simulink model "MRAS_SMC_SFOC_1_5KW_15May21"  (R2017b)
settings: Solver=FixedStepDiscrete  StartTime=0.0  StopTime=3  FixedStep=Tsim  MaxStep=1e-6  RelTol=1e-3
values from neighbouring files (symbols this model uses):
  F = 1e-20    [ParametreMRAS_SMC_SFOC_1_5KW.m]
  Jm = 0.076    [ParametreMRAS_SMC_SFOC_1_5KW.m]
  Lm = 0.3032    [ParametreMRAS_SMC_SFOC_1_5KW.m]
  Lr = Lm+Lls    (= 0.32009)    [ParametreMRAS_SMC_SFOC_1_5KW.m]
  Ls = Lm+Llr    (= 0.32009)    [ParametreMRAS_SMC_SFOC_1_5KW.m]
  M = 0.3032    [ParametreMRAS_SMC_SFOC_1_5KW.m]
  Npole = 2    [ParametreMRAS_SMC_SFOC_1_5KW.m]
  Rr = 4.75    [ParametreMRAS_SMC_SFOC_1_5KW.m]
  Rs = 4.74    [ParametreMRAS_SMC_SFOC_1_5KW.m]
  sig = 1-((M^2)/(Ls*Lr))    (= 0.102748524929)    [ParametreMRAS_SMC_SFOC_1_5KW.m]
  T2_3 = T3_2'    [ParametreMRAS_SMC_SFOC_1_5KW.m]
  T3_2 = sqrt(2/3)*[cos(0) cos(2*pi/3) cos(4*pi/3);sin(0) sin(2*pi/3) sin(4*pi/3)]    [ParametreMRAS_SMC_SFOC_1_5KW.m]
  Tr = Lr/Rr    (= 0.0673873684211)    [ParametreMRAS_SMC_SFOC_1_5KW.m]
  Tsim = 0.5e-5    (= 5e-06)    [ParametreMRAS_SMC_SFOC_1_5KW.m]
  Tss = Ls/Rs    (= 0.067529535865)    [ParametreMRAS_SMC_SFOC_1_5KW.m]
undefined symbols (not defined in the file or in its folder): DiscIntNeverNeededParam
libraries: simulink x1
settings Model: Creator=momo  LastModifiedBy=LENOVO

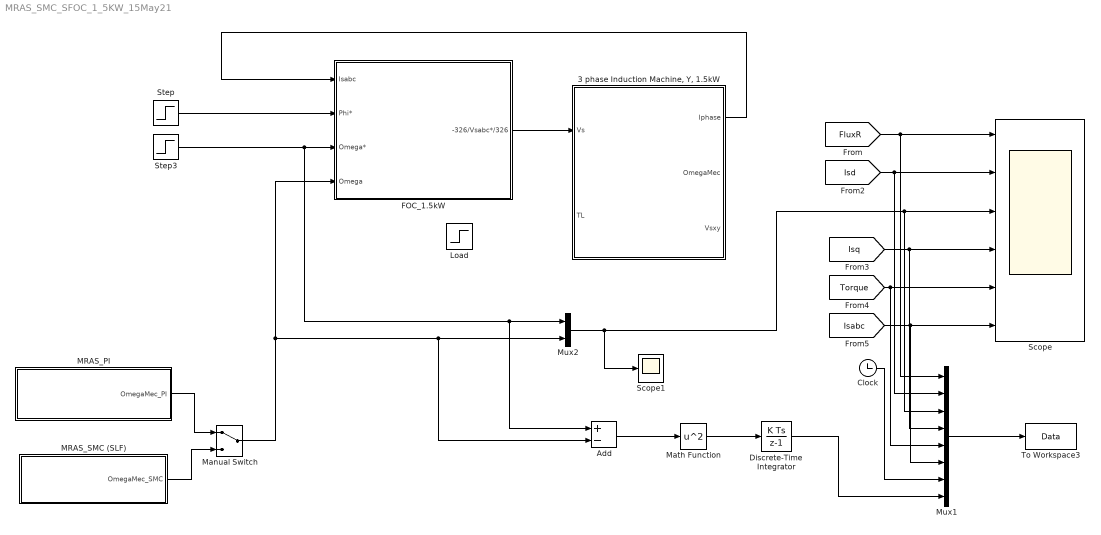
== system MRAS_SMC_SFOC_1_5KW_15May21 ==
  "3 phase Induction Machine, Y, 1.5kW" : Subsystem
  Add : Sum  Inputs=+-
  Clock : Clock
      settings: Decimation=100
  Discrete-Time Integrator : DiscreteIntegrator  InitialConditionSetting=State (most efficient)  SampleTime=-1  ICPrevOutput=DiscIntNeverNeededParam  ICPrevScaledInput=DiscIntNeverNeededParam
  FOC_1.5kW : Subsystem
  Load : Step  After=36.22  SampleTime=Tsim
  MRAS_PI : Subsystem
  MRAS_SMC (SLF) : Subsystem
  Manual Switch : ManualSwitch
  Math Function : Math  Operator=square  SaturateOnIntegerOverflow=on
  Mux1 : Mux  Inputs=8
  Mux2 : Mux  Inputs=2
  Scope : Scope  NumInputPorts=6
  Scope1 : Scope
  Step : Step  Time=0  After=1.2  SampleTime=Tsim
  Step3 : Step  Time=0.3  After=50  SampleTime=0
  To Workspace3 : ToWorkspace  VariableName=Data  SampleTime=-1
  wires:
  "3 phase Induction Machine, Y, 1.5kW"/1(Iphase) -> FOC_1.5kW/1(Isabc)
  Step/1 -> FOC_1.5kW/2(Phi*)
  [FluxR] -> Mux1/1, Scope/1
  [Isd] -> Mux1/2, Scope/2
  Mux2/1 -> Mux1/3, Scope/3, Scope1/1
  [Isq] -> Mux1/4, Scope/4
  [Torque] -> Mux1/5, Scope/5
  [Isabc] -> Mux1/6, Scope/6
  FOC_1.5kW/1(-326/Vsabc*/326) -> "3 phase Induction Machine, Y, 1.5kW"/1(Vs)
  Add/1 -> Math Function/1
  Math Function/1 -> Discrete-Time Integrator/1
  Step3/1 -> FOC_1.5kW/3(Omega*), Add/1, Mux2/1
  Manual Switch/1 -> Add/2, Mux2/2, FOC_1.5kW/4(Omega)
  Clock/1 -> Mux1/7
  Discrete-Time Integrator/1 -> Mux1/8
  Mux1/1 -> To Workspace3/1
  MRAS_SMC (SLF)/1(OmegaMec_SMC) -> Manual Switch/2
  MRAS_PI/1(OmegaMec_PI) -> Manual Switch/1

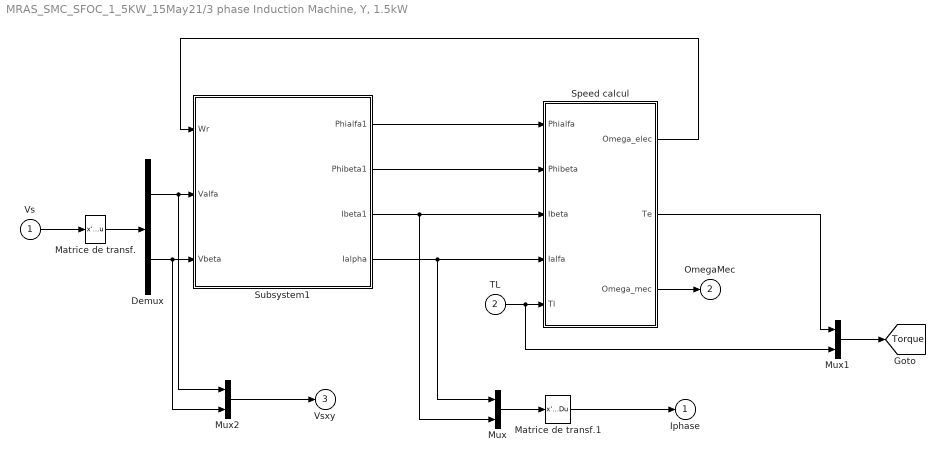
== system MRAS_SMC_SFOC_1_5KW_15May21/3 phase Induction Machine, Y, 1.5kW ==
  Vs : Inport
  TL : Inport  Port=2
  Demux : Demux  Outputs=2
  Matrice de transf. : StateSpace  A=[]  B=[]  C=[]  D=K  InitialCondition=0  mask(Matrix Gain){K=T3_2}
      mask prompts: K "Gain matrix:"
      mask help: Matrix Gain.
      mask Help: Multiplies input vector by entered matrix to produce output vector (y=Au).
      mask Display: disp('K')
  Matrice de transf.1 : StateSpace  A=[]  B=[]  C=[]  D=K  InitialCondition=0  mask(Matrix Gain){K=T2_3}
      mask prompts: K "Gain matrix:"
      mask help: Matrix Gain.
      mask Help: Multiplies input vector by entered matrix to produce output vector (y=Au).
      mask Display: disp('K')
  Mux : Mux  Inputs=2
  Mux1 : Mux  Inputs=2
  Mux2 : Mux  Inputs=2
  Speed calcul : Subsystem
  Subsystem1 : Subsystem
  Iphase : Outport  InitialOutput=0
  OmegaMec : Outport  Port=2  InitialOutput=0
  Vsxy : Outport  Port=3  InitialOutput=0
  tag scope: Torque=global
  wires:
  Subsystem1/3(Ibeta1) -> Speed calcul/3(Ibeta), Mux/2
  Subsystem1/4(Ialpha) -> Speed calcul/4(Ialfa), Mux/1
  Speed calcul/3(Omega_mec) -> OmegaMec/1
  Mux/1 -> Matrice de transf.1/1
  Matrice de transf./1 -> Demux/1
  Demux/2 -> Mux2/2, Subsystem1/3(Vbeta)
  Demux/1 -> Mux2/1, Subsystem1/2(Valfa)
  Subsystem1/2(Phibeta1) -> Speed calcul/2(Phibeta)
  Subsystem1/1(Phialfa1) -> Speed calcul/1(Phialfa)
  TL/1 -> Mux1/2, Speed calcul/5(Tl)
  Vs/1 -> Matrice de transf./1
  Matrice de transf.1/1 -> Iphase/1
  Speed calcul/1(Omega_elec) -> Subsystem1/1(Wr)
  Speed calcul/2(Te) -> Mux1/1
  Mux1/1 -> [Torque]
  Mux2/1 -> Vsxy/1

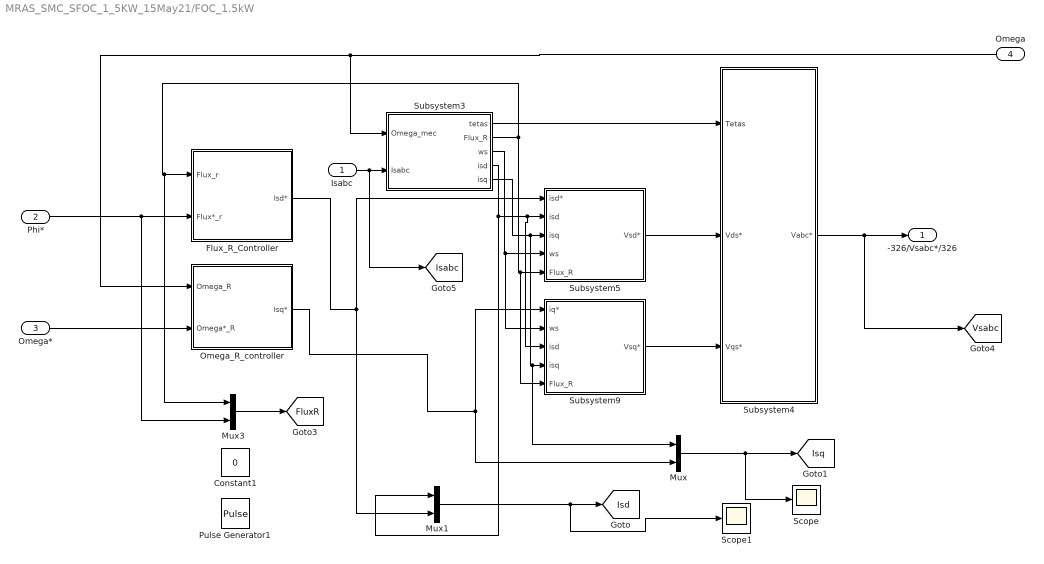
== system MRAS_SMC_SFOC_1_5KW_15May21/FOC_1.5kW ==
  Isabc : Inport
  Phi* : Inport  Port=2
  Omega* : Inport  Port=3
  Omega : Inport  Port=4
  Constant1 : Constant  Value=0
  Flux_R_Controller : Subsystem
  Mux : Mux  Inputs=2
  Mux1 : Mux  Inputs=2
  Mux3 : Mux  Inputs=2
  Omega_R_controller : Subsystem
  Pulse Generator1 : DiscretePulseGenerator  PulseType=Time based  Period=0.5  PulseWidth=50
  Scope : Scope
  Scope1 : Scope
  Subsystem3 : Subsystem
  Subsystem4 : Subsystem
  Subsystem5 : Subsystem
  Subsystem9 : Subsystem
  -326/Vsabc*/326 : Outport
  tag scope: FluxR=global, Isabc=global, Isd=global, Isq=global, Vsabc=global
  wires:
  Subsystem4/1(Vabc*) -> [Vsabc], -326/Vsabc*/326/1
  Omega/1 -> Omega_R_controller/1(Omega_R), Subsystem3/1(Omega_mec)
  Omega*/1 -> Omega_R_controller/2(Omega*_R)
  Isabc/1 -> [Isabc], Subsystem3/2(Isabc)
  Mux/1 -> Scope/1, [Isq]
  Mux1/1 -> Scope1/1, [Isd]
  Subsystem5/1(Vsd*) -> Subsystem4/2(Vds*)
  Subsystem9/1(Vsq*) -> Subsystem4/3(Vqs*)
  Phi*/1 -> Mux3/2, Flux_R_Controller/2(Flux*_r)
  Subsystem3/1(tetas) -> Subsystem4/1(Tetas)
  Subsystem3/3(ws) -> Subsystem9/2(ws), Subsystem5/4(ws)
  Subsystem3/4(isd) -> Mux1/1, Subsystem9/3(isd), Subsystem5/2(isd)
  Subsystem3/5(isq) -> Mux/1, Subsystem9/4(isq), Subsystem5/3(isq)
  Subsystem3/2(Flux_R) -> Subsystem9/5(Flux_R), Subsystem5/5(Flux_R), Mux3/1, Flux_R_Controller/1(Flux_r)
  Mux3/1 -> [FluxR]
  Omega_R_controller/1(Isq*) -> Mux/2, Subsystem9/1(iq*)
  Flux_R_Controller/1(Isd*) -> Mux1/2, Subsystem5/1(isd*)

== system MRAS_SMC_SFOC_1_5KW_15May21/MRAS_PI ==
  Gain1 : Gain  Gain=60/2/pi/2
  PI : simulink/Continuous/PID Controller  Controller=PID  TimeDomain=Discrete-time  SampleTime=Tsim  IntegratorMethod=Forward Euler  FilterMethod=Forward Euler  Form=Parallel  UseFilter=on  ControllerParametersSource=internal  P=200  I=4000  D=0  N=100  InitialConditionSource=internal  InitialConditionForIntegrator=0  InitialConditionForFilter=0  ExternalReset=none  LimitOutput=on  UpperSaturationLimit=400  LowerSaturationLimit=-400  LinearizeAsGain=off  AntiWindupMode=none  Kb=1  TrackingMode=off  Kt=1  PParamMin=[]  PParamMax=[]  IParamMin=[]  IParamMax=[]  DParamMin=[]  DParamMax=[]  NParamMin=[]  NParamMax=[]  KbParamMin=[]  KbParamMax=[]  KtParamMin=[]  KtParamMax=[]  POutMin=[]  POutMax=[]  IOutMin=[]  IOutMax=[]  DOutMin=[]  DOutMax=[]  NOutMin=[]  NOutMax=[]  KbOutMin=[]  KbOutMax=[]  KtOutMin=[]  KtOutMax=[]  IntegratorOutMin=[]  IntegratorOutMax=[]  FilterOutMin=[]  FilterOutMax=[]  SumOutMin=[]  SumOutMax=[]  SumI1OutMin=[]  SumI1OutMax=[]  SumI2OutMin=[]  SumI2OutMax=[]  SumI3OutMin=[]  SumI3OutMax=[]  SumDOutMin=[]  SumDOutMax=[]  SaturationOutMin=[]  SaturationOutMax=[]  IntegratorContinuousStateAttributes=''  IntegratorStateMustResolveToSignalObject=off  IntegratorRTWStateStorageClass=Auto  FilterContinuousStateAttributes=''  FilterStateMustResolveToSignalObject=off  FilterRTWStateStorageClass=Auto  DifferentiatorICPrevScaledInput=0  DifferentiatorOutMin=[]  DifferentiatorOutMax=[]  InitialConditionSetting=State (most efficient)  FilterDiffOutCoefMin=[]  FilterDiffOutCoefMax=[]  SumDenOutMin=[]  SumDenOutMax=[]  SumNumOutMin=[]  SumNumOutMax=[]  ReciprocalOutMin=[]  ReciprocalOutMax=[]  DivideOutMin=[]  DivideOutMax=[]  TunerSelectOption=Transfer Function Based (PID Tuner App)
  Product1 : Product  RndMeth=Zero
  Product2 : Product  RndMeth=Zero
  Subsystem1 : Subsystem
  Subtract1 : Sum  Inputs=-+
  OmegaMec_PI : Outport
  wires:
  Subtract1/1 -> PI/1
  PI/1 -> Gain1/1, Subsystem1/3(wr)
  Product2/1 -> Subtract1/2
  Product1/1 -> Subtract1/1
  [Vsabc] -> Subsystem1/2(Vphase)
  [Isabc] -> Subsystem1/1(iphase)
  Subsystem1/3(phi_r_al_esti) -> Product2/2
  Subsystem1/2(phi_r_beta_ref) -> Product2/1
  Subsystem1/4(phi_r_beta_estim) -> Product1/2
  Subsystem1/1(phi_r_al_ref) -> Product1/1
  Gain1/1 -> OmegaMec_PI/1

== system MRAS_SMC_SFOC_1_5KW_15May21/MRAS_SMC (SLF) ==
  Gain1 : Gain  Gain=60/2/pi/2
  Product1 : Product  RndMeth=Zero
  Product2 : Product  RndMeth=Zero
  Subsystem1 : Subsystem
  Subsystem6 : Subsystem
  Subtract1 : Sum  Inputs=-+
  OmegaMec_SMC : Outport
  wires:
  [Vsabc] -> Subsystem1/2(Vphase)
  [Isabc] -> Subsystem1/1(iphase)
  Gain1/1 -> OmegaMec_SMC/1
  Subtract1/1 -> Subsystem6/1(Error)
  Subsystem6/1(Wm) -> Gain1/1, Subsystem1/3(wr)
  Product2/1 -> Subtract1/2
  Product1/1 -> Subtract1/1
  Subsystem1/3(phi_r_al_esti) -> Product2/2
  Subsystem1/2(phi_r_beta_ref) -> Product2/1
  Subsystem1/4(phi_r_beta_estim) -> Product1/2
  Subsystem1/1(phi_r_al_ref) -> Product1/1

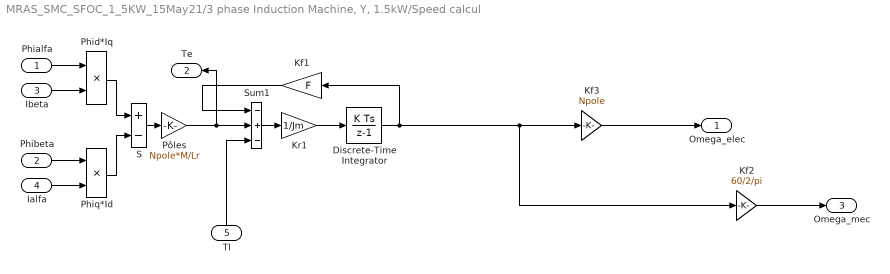
== system MRAS_SMC_SFOC_1_5KW_15May21/3 phase Induction Machine, Y, 1.5kW/Speed calcul ==
  Phialfa : Inport
  Phibeta : Inport  Port=2
  Ibeta : Inport  Port=3
  Ialfa : Inport  Port=4
  Tl : Inport  Port=5
  Discrete-Time Integrator : DiscreteIntegrator  InitialConditionSetting=State (most efficient)  SampleTime=Tsim  ICPrevOutput=DiscIntNeverNeededParam  ICPrevScaledInput=DiscIntNeverNeededParam
  Kf1 : Gain  Gain=F  OutDataTypeStr=Inherit: Same as input  ParamDataTypeStr=Inherit: Same as input
  Kf2 : Gain  Gain=60/2/pi  SaturateOnIntegerOverflow=on  OutDataTypeStr=Inherit: Same as input  ParamDataTypeStr=Inherit: Same as input
  Kf3 : Gain  Gain=Npole  SaturateOnIntegerOverflow=on  OutDataTypeStr=Inherit: Same as input  ParamDataTypeStr=Inherit: Same as input
  Kr1 : Gain  Gain=1/Jm  OutDataTypeStr=Inherit: Same as input  ParamDataTypeStr=Inherit: Same as input
  Phid*Iq : Product  SaturateOnIntegerOverflow=on  RndMeth=Zero  InputSameDT=on  OutDataTypeStr=Inherit: Same as first input
  Phiq*Id : Product  SaturateOnIntegerOverflow=on  RndMeth=Zero  InputSameDT=on  OutDataTypeStr=Inherit: Same as first input
  Pôles : Gain  Gain=Npole*M/Lr  SaturateOnIntegerOverflow=on  OutDataTypeStr=Inherit: Same as input  ParamDataTypeStr=Inherit: Same as input
  S : Sum  Inputs=+-  SaturateOnIntegerOverflow=on  InputSameDT=on  OutDataTypeStr=Inherit: Same as first input
  Sum1 : Sum  Inputs=-+-  InputSameDT=on  OutDataTypeStr=Inherit: Same as first input
  Omega_elec : Outport
  Te : Outport  Port=2
  Omega_mec : Outport  Port=3
  wires:
  Kf2/1 -> Omega_mec/1
  Tl/1 -> Sum1/3
  Phibeta/1 -> Phiq*Id/1
  Kf3/1 -> Omega_elec/1
  Ialfa/1 -> Phiq*Id/2
  Ibeta/1 -> Phid*Iq/2
  Phialfa/1 -> Phid*Iq/1
  Phiq*Id/1 -> S/2
  Phid*Iq/1 -> S/1
  Discrete-Time Integrator/1 -> Kf3/1, Kf2/1, Kf1/1
  Kr1/1 -> Discrete-Time Integrator/1
  Sum1/1 -> Kr1/1
  Pôles/1 -> Te/1, Sum1/2
  S/1 -> Pôles/1
  Kf1/1 -> Sum1/1

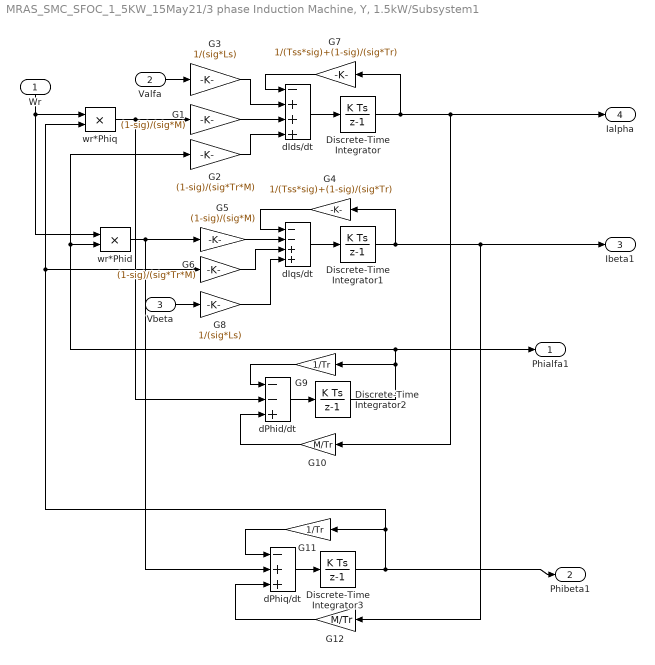
== system MRAS_SMC_SFOC_1_5KW_15May21/3 phase Induction Machine, Y, 1.5kW/Subsystem1 ==
  Wr : Inport
  Valfa : Inport  Port=2
  Vbeta : Inport  Port=3
  Discrete-Time Integrator{,1..3} (4 alike) : DiscreteIntegrator  InitialConditionSetting=State (most efficient)  SampleTime=Tsim  ICPrevOutput=DiscIntNeverNeededParam  ICPrevScaledInput=DiscIntNeverNeededParam
  G1 : Gain  Gain=(1-sig)/(sig*M)  SaturateOnIntegerOverflow=on  OutDataTypeStr=Inherit: Same as input  ParamDataTypeStr=Inherit: Same as input
  G10 : Gain  Gain=M/Tr  SaturateOnIntegerOverflow=on  OutDataTypeStr=Inherit: Same as input  ParamDataTypeStr=Inherit: Same as input
  G11 : Gain  Gain=1/Tr  SaturateOnIntegerOverflow=on  OutDataTypeStr=Inherit: Same as input  ParamDataTypeStr=Inherit: Same as input
  G12 : Gain  Gain=M/Tr  SaturateOnIntegerOverflow=on  OutDataTypeStr=Inherit: Same as input  ParamDataTypeStr=Inherit: Same as input
  G2 : Gain  Gain=(1-sig)/(sig*Tr*M)  SaturateOnIntegerOverflow=on  OutDataTypeStr=Inherit: Same as input  ParamDataTypeStr=Inherit: Same as input
  G3 : Gain  Gain=1/(sig*Ls)  SaturateOnIntegerOverflow=on  OutDataTypeStr=Inherit: Same as input  ParamDataTypeStr=Inherit: Same as input
  G4 : Gain  Gain=1/(Tss*sig)+(1-sig)/(sig*Tr)  SaturateOnIntegerOverflow=on  OutDataTypeStr=Inherit: Same as input  ParamDataTypeStr=Inherit: Same as input
  G5 : Gain  Gain=(1-sig)/(sig*M)  SaturateOnIntegerOverflow=on  OutDataTypeStr=Inherit: Same as input  ParamDataTypeStr=Inherit: Same as input
  G6 : Gain  Gain=(1-sig)/(sig*Tr*M)  SaturateOnIntegerOverflow=on  OutDataTypeStr=Inherit: Same as input  ParamDataTypeStr=Inherit: Same as input
  G7 : Gain  Gain=1/(Tss*sig)+(1-sig)/(sig*Tr)  SaturateOnIntegerOverflow=on  OutDataTypeStr=Inherit: Same as input  ParamDataTypeStr=Inherit: Same as input
  G8 : Gain  Gain=1/(sig*Ls)  SaturateOnIntegerOverflow=on  OutDataTypeStr=Inherit: Same as input  ParamDataTypeStr=Inherit: Same as input
  G9 : Gain  Gain=1/Tr  SaturateOnIntegerOverflow=on  OutDataTypeStr=Inherit: Same as input  ParamDataTypeStr=Inherit: Same as input
  dIds/dt : Sum  Inputs=-+++  SaturateOnIntegerOverflow=on  InputSameDT=on  OutDataTypeStr=Inherit: Same as first input
  dIqs/dt : Sum  Inputs=--++  SaturateOnIntegerOverflow=on  InputSameDT=on  OutDataTypeStr=Inherit: Same as first input
  dPhid/dt : Sum  Inputs=--+  SaturateOnIntegerOverflow=on  InputSameDT=on  OutDataTypeStr=Inherit: Same as first input
  dPhiq/dt : Sum  Inputs=-++  SaturateOnIntegerOverflow=on  InputSameDT=on  OutDataTypeStr=Inherit: Same as first input
  wr*Phid : Product  SaturateOnIntegerOverflow=on  RndMeth=Zero  InputSameDT=on  OutDataTypeStr=Inherit: Same as first input
  wr*Phiq : Product  SaturateOnIntegerOverflow=on  RndMeth=Zero  InputSameDT=on  OutDataTypeStr=Inherit: Same as first input
  Phialfa1 : Outport
  Phibeta1 : Outport  Port=2
  Ibeta1 : Outport  Port=3
  Ialpha : Outport  Port=4
  wires:
  Vbeta/1 -> G8/1
  Valfa/1 -> G3/1
  Wr/1 -> wr*Phiq/1, wr*Phid/1
  dIds/dt/1 -> Discrete-Time Integrator/1
  Discrete-Time Integrator/1 -> G10/1, Ialpha/1, G7/1
  G7/1 -> dIds/dt/1
  G1/1 -> dIds/dt/3
  G3/1 -> dIds/dt/2
  G2/1 -> dIds/dt/4
  dPhid/dt/1 -> Discrete-Time Integrator2/1
  Discrete-Time Integrator2/1 -> G9/1, Phialfa1/1, G2/1, wr*Phid/2
  G9/1 -> dPhid/dt/1
  G10/1 -> dPhid/dt/3
  G11/1 -> dPhiq/dt/1
  G12/1 -> dPhiq/dt/3
  G8/1 -> dIqs/dt/4
  G6/1 -> dIqs/dt/3
  G5/1 -> dIqs/dt/2
  wr*Phid/1 -> G5/1, dPhiq/dt/2
  G4/1 -> dIqs/dt/1
  Discrete-Time Integrator1/1 -> G12/1, Ibeta1/1, G4/1
  wr*Phiq/1 -> G1/1, dPhid/dt/2
  Discrete-Time Integrator3/1 -> G6/1, wr*Phiq/2, G11/1, Phibeta1/1
  dPhiq/dt/1 -> Discrete-Time Integrator3/1
  dIqs/dt/1 -> Discrete-Time Integrator1/1

== system MRAS_SMC_SFOC_1_5KW_15May21/FOC_1.5kW/Flux_R_Controller ==
  Flux_r : Inport
  Flux*_r : Inport  Port=2
  -5<isd*<5 : Saturate  UpperLimit=5  LowerLimit=-5
  Add1 : Sum  Inputs=-+
  Add2 : Sum
  Gain : Gain  Gain=1000
  Gain1 : Gain  Gain=100
  Saturated_Integrator : DiscreteIntegrator  InitialConditionSetting=State (most efficient)  SampleTime=Tsim  LimitOutput=on  UpperSaturationLimit=5  LowerSaturationLimit=-5  ICPrevOutput=DiscIntNeverNeededParam  ICPrevScaledInput=DiscIntNeverNeededParam
  Scope : Scope
  Isd* : Outport
  wires:
  Gain/1 -> Saturated_Integrator/1
  Gain1/1 -> Add2/2
  Add2/1 -> -5<isd*<5/1
  Saturated_Integrator/1 -> Scope/1, Add2/1
  -5<isd*<5/1 -> Isd*/1
  Flux_r/1 -> Add1/1
  Flux*_r/1 -> Add1/2
  Add1/1 -> Gain1/1, Gain/1

== system MRAS_SMC_SFOC_1_5KW_15May21/FOC_1.5kW/Omega_R_controller ==
  Omega_R : Inport
  Omega*_R : Inport  Port=2
  -5<isq*<5 : Saturate  UpperLimit=5  LowerLimit=-5
  Add : Sum  Inputs=-+
  Add2 : Sum
  Discrete-Time Integrator : DiscreteIntegrator  InitialConditionSetting=State (most efficient)  SampleTime=Tsim  LimitOutput=on  UpperSaturationLimit=5  LowerSaturationLimit=-5  ICPrevOutput=DiscIntNeverNeededParam  ICPrevScaledInput=DiscIntNeverNeededParam
  Gain1 : Gain  Gain=10
  Gain3 : Gain  Gain=0
  Gain4 : Gain  Gain=100
  Kf1 : Gain  Gain=2*pi/60  SaturateOnIntegerOverflow=on  OutDataTypeStr=Inherit: Same as input  ParamDataTypeStr=Inherit: Same as input
  Scope : Scope
  Isq* : Outport
  wires:
  -5<isq*<5/1 -> Scope/1, Isq*/1
  Discrete-Time Integrator/1 -> Add2/1
  Add2/1 -> -5<isq*<5/1
  Gain1/1 -> Add2/2
  Gain3/1 -> Discrete-Time Integrator/1
  Omega*_R/1 -> Add/2
  Omega_R/1 -> Add/1
  Add/1 -> Kf1/1
  Kf1/1 -> Gain3/1, Gain1/1

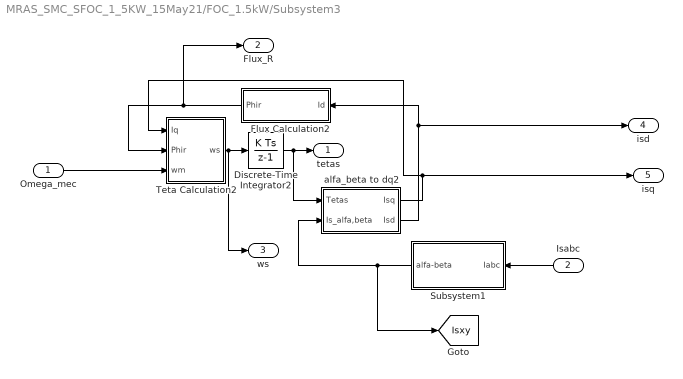
== system MRAS_SMC_SFOC_1_5KW_15May21/FOC_1.5kW/Subsystem3 ==
  Omega_mec : Inport
  Isabc : Inport  Port=2
  Discrete-Time Integrator2 : DiscreteIntegrator  InitialConditionSetting=State (most efficient)  SampleTime=Tsim  ICPrevOutput=DiscIntNeverNeededParam  ICPrevScaledInput=DiscIntNeverNeededParam
  Flux Calculation2 : Subsystem  mask(Flux Calcultation){}
      mask init:
      | NF=0.44572610323020e-6;
      | DF=[1 -0.99998715486734];
      mask Display: disp('Flux\nCalc.')
  Subsystem1 : Subsystem
  Teta Calculation2 : Subsystem
  alfa_beta to dq2 : Subsystem
  tetas : Outport
  Flux_R : Outport  Port=2
  ws : Outport  Port=3
  isd : Outport  Port=4
  isq : Outport  Port=5
  tag scope: Isxy=global
  wires:
  Teta Calculation2/1(ws) -> Discrete-Time Integrator2/1, ws/1
  alfa_beta to dq2/1(Isq) -> Teta Calculation2/1(Iq), isq/1
  alfa_beta to dq2/2(Isd) -> Flux Calculation2/1(Id), isd/1
  Discrete-Time Integrator2/1 -> tetas/1, alfa_beta to dq2/1(Tetas)
  Flux Calculation2/1(Phir) -> Teta Calculation2/2(Phir), Flux_R/1
  Subsystem1/1(alfa-beta) -> [Isxy], alfa_beta to dq2/2(Is_alfa,beta)
  Isabc/1 -> Subsystem1/1(Iabc)
  Omega_mec/1 -> Teta Calculation2/3(wm)

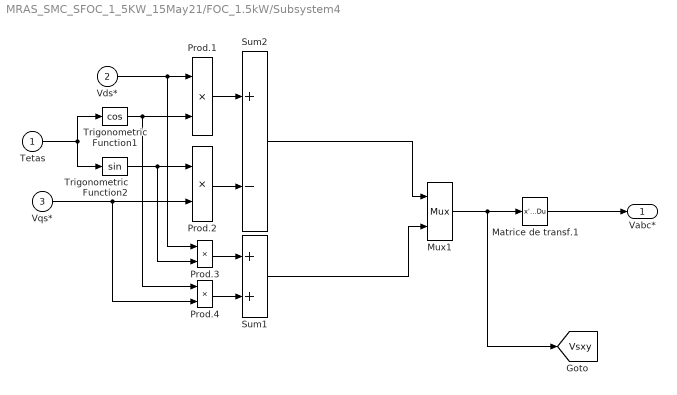
== system MRAS_SMC_SFOC_1_5KW_15May21/FOC_1.5kW/Subsystem4 ==
  Tetas : Inport
  Vds* : Inport  Port=2
  Vqs* : Inport  Port=3
  Matrice de transf.1 : StateSpace  A=[]  B=[]  C=[]  D=K  InitialCondition=0  mask(Matrix Gain){K=T2_3}
      mask prompts: K "Gain matrix:"
      mask help: Matrix Gain.
      mask Help: Multiplies input vector by entered matrix to produce output vector (y=Au).
      mask Display: disp('K')
  Mux1 : Mux  Inputs=2
  Prod.{1..4} (4 alike) : Product  SaturateOnIntegerOverflow=on  InputSameDT=on  OutDataTypeStr=Inherit: Same as first input
  Sum1 : Sum  SaturateOnIntegerOverflow=on  InputSameDT=on  OutDataTypeStr=Inherit: Same as first input
  Sum2 : Sum  Inputs=+-  SaturateOnIntegerOverflow=on  InputSameDT=on  OutDataTypeStr=Inherit: Same as first input
  Trigonometric Function1 : Trigonometry  Operator=cos
  Trigonometric Function2 : Trigonometry
  Vabc* : Outport
  tag scope: Vsxy=global
  wires:
  Tetas/1 -> Trigonometric Function1/1, Trigonometric Function2/1
  Prod.4/1 -> Sum1/2
  Prod.3/1 -> Sum1/1
  Vqs*/1 -> Prod.2/2, Prod.4/2
  Vds*/1 -> Prod.1/1, Prod.3/1
  Prod.2/1 -> Sum2/2
  Prod.1/1 -> Sum2/1
  Trigonometric Function2/1 -> Prod.3/2, Prod.2/1
  Trigonometric Function1/1 -> Prod.4/1, Prod.1/2
  Mux1/1 -> [Vsxy], Matrice de transf.1/1
  Sum1/1 -> Mux1/2
  Matrice de transf.1/1 -> Vabc*/1
  Sum2/1 -> Mux1/1

== system MRAS_SMC_SFOC_1_5KW_15May21/FOC_1.5kW/Subsystem5 ==
  isd* : Inport
  isd : Inport  Port=2
  isq : Inport  Port=3
  ws : Inport  Port=4
  Flux_R : Inport  Port=5
  -400<Vsd*<400 : Saturate  UpperLimit=400  LowerLimit=-400
  Add : Sum  Inputs=-+
  Add4 : Sum  Inputs=+-
  Mux2 : Mux  Inputs=3
  d-Current controller : Subsystem
  femd : Fcn  Expr=u(3)*sig*Ls*u(1)+(M/Lr^2)*Rr*u(2)
  Vsd* : Outport  InitialOutput=0
  wires:
  isd/1 -> Add/1
  isd*/1 -> Add/2
  Mux2/1 -> femd/1
  isq/1 -> Mux2/1
  ws/1 -> Mux2/3
  Flux_R/1 -> Mux2/2
  Add4/1 -> -400<Vsd*<400/1
  -400<Vsd*<400/1 -> Vsd*/1
  femd/1 -> Add4/2
  Add/1 -> d-Current controller/1(Error Isd)
  d-Current controller/1(Vsd*) -> Add4/1

== system MRAS_SMC_SFOC_1_5KW_15May21/FOC_1.5kW/Subsystem9 ==
  iq* : Inport
  ws : Inport  Port=2
  isd : Inport  Port=3
  isq : Inport  Port=4
  Flux_R : Inport  Port=5
  -400<V*sq<400 : Saturate  UpperLimit=400  LowerLimit=-400
  Add : Sum  Inputs=-+
  Add3 : Sum  Inputs=+-
  Fcn1 : Fcn  Expr=-u(4)*sig*Ls*u(1)-u(4)*(M/Lr)*u(3)+(M^2/Lr/Tr)*u(2)
  Mux1 : Mux
  q-Current controller : Subsystem
  Vsq* : Outport  InitialOutput=0
  wires:
  Mux1/1 -> Fcn1/1
  ws/1 -> Mux1/4
  isd/1 -> Mux1/1
  Flux_R/1 -> Mux1/3
  isq/1 -> Mux1/2, Add/1
  iq*/1 -> Add/2
  Add3/1 -> -400<V*sq<400/1
  -400<V*sq<400/1 -> Vsq*/1
  Fcn1/1 -> Add3/2
  Add/1 -> q-Current controller/1(Error Isq)
  q-Current controller/1(Vsq*) -> Add3/1

== system MRAS_SMC_SFOC_1_5KW_15May21/MRAS_PI/Subsystem1 ==
  iphase : Inport
  Vphase : Inport  Port=2
  wr : Inport  Port=3
  Subsystem : Subsystem
  model reference : Subsystem
  phi_r_al_ref : Outport
  phi_r_beta_ref : Outport  Port=2
  phi_r_al_esti : Outport  Port=3
  phi_r_beta_estim : Outport  Port=4
  wires:
  model reference/2(phi_r_bet_ref) -> phi_r_beta_ref/1
  model reference/1(phi_r_al_ref) -> phi_r_al_ref/1
  iphase/1 -> model reference/1(Iaa'bb'cc')
  Vphase/1 -> model reference/2(Vaa'bb'cc')
  Subsystem/2(PhirBeta) -> phi_r_beta_estim/1
  Subsystem/1(Phiralpha) -> phi_r_al_esti/1
  model reference/3(Isal) -> Subsystem/1(Isalpha)
  model reference/4(Isbeta) -> Subsystem/2(Isbeta)
  wr/1 -> Subsystem/3(In3)

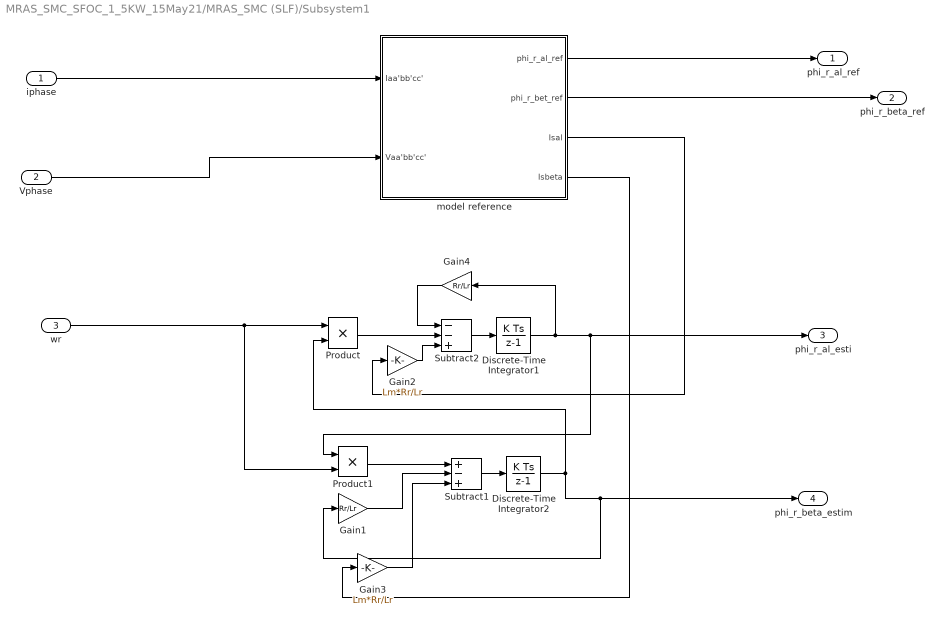
== system MRAS_SMC_SFOC_1_5KW_15May21/MRAS_SMC (SLF)/Subsystem1 ==
  iphase : Inport
  Vphase : Inport  Port=2
  wr : Inport  Port=3
  Discrete-Time Integrator1 : DiscreteIntegrator  InitialConditionSetting=State (most efficient)  SampleTime=Tsim  ICPrevOutput=DiscIntNeverNeededParam  ICPrevScaledInput=DiscIntNeverNeededParam
  Discrete-Time Integrator2 : DiscreteIntegrator  InitialConditionSetting=State (most efficient)  SampleTime=Tsim  ICPrevOutput=DiscIntNeverNeededParam  ICPrevScaledInput=DiscIntNeverNeededParam
  Gain1 : Gain  Gain=Rr/Lr
  Gain2 : Gain  Gain=Lm*Rr/Lr
  Gain3 : Gain  Gain=Lm*Rr/Lr
  Gain4 : Gain  Gain=Rr/Lr
  Product : Product  RndMeth=Zero
  Product1 : Product  RndMeth=Zero
  Subtract1 : Sum  Inputs=+-+
  Subtract2 : Sum  Inputs=--+
  model reference : Subsystem
  phi_r_al_ref : Outport
  phi_r_beta_ref : Outport  Port=2
  phi_r_al_esti : Outport  Port=3
  phi_r_beta_estim : Outport  Port=4
  wires:
  Subtract2/1 -> Discrete-Time Integrator1/1
  Discrete-Time Integrator1/1 -> phi_r_al_esti/1, Product1/1, Gain4/1
  Vphase/1 -> model reference/2(Vaa'bb'cc')
  iphase/1 -> model reference/1(Iaa'bb'cc')
  model reference/1(phi_r_al_ref) -> phi_r_al_ref/1
  model reference/2(phi_r_bet_ref) -> phi_r_beta_ref/1
  Subtract1/1 -> Discrete-Time Integrator2/1
  Discrete-Time Integrator2/1 -> Product/2, phi_r_beta_estim/1, Gain1/1
  Product/1 -> Subtract2/2
  wr/1 -> Product/1, Product1/2
  Product1/1 -> Subtract1/1
  Gain2/1 -> Subtract2/3
  Gain3/1 -> Subtract1/3
  Gain4/1 -> Subtract2/1
  Gain1/1 -> Subtract1/2
  model reference/4(Isbeta) -> Gain3/1
  model reference/3(Isal) -> Gain2/1

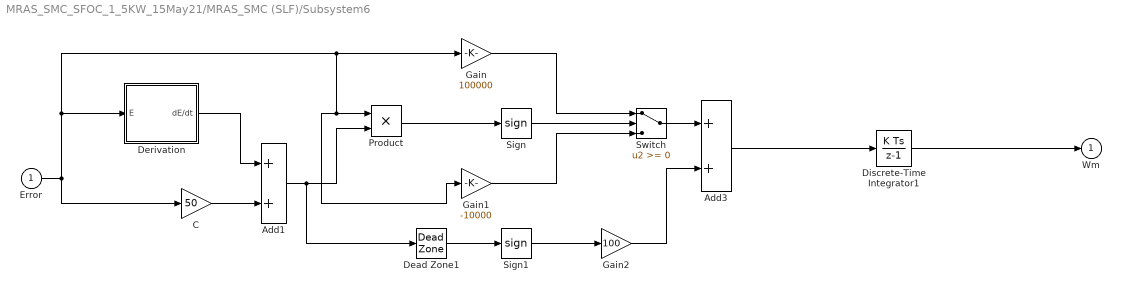
== system MRAS_SMC_SFOC_1_5KW_15May21/MRAS_SMC (SLF)/Subsystem6 ==
  Error : Inport
  Add1 : Sum
  Add3 : Sum
  C : Gain  Gain=50
  Dead Zone1 : DeadZone  LowerValue=-.3  UpperValue=.3  SaturateOnIntegerOverflow=on
  Derivation : Subsystem
  Discrete-Time Integrator1 : DiscreteIntegrator  InitialConditionSetting=State (most efficient)  SampleTime=Tsim  ICPrevOutput=DiscIntNeverNeededParam  ICPrevScaledInput=DiscIntNeverNeededParam
  Gain : Gain  Gain=100000
  Gain1 : Gain  Gain=-10000
  Gain2 : Gain  Gain=100
  Product : Product  RndMeth=Zero
  Sign : Signum
  Sign1 : Signum  ZeroCross=off
  Switch : Switch
  Wm : Outport  InitialOutput=0
  wires:
  Gain2/1 -> Add3/2
  Dead Zone1/1 -> Sign1/1
  Derivation/1(dE/dt) -> Add1/1
  Discrete-Time Integrator1/1 -> Wm/1
  Add1/1 -> Product/2, Dead Zone1/1
  Sign1/1 -> Gain2/1
  Gain1/1 -> Switch/3
  Gain/1 -> Switch/1
  Add3/1 -> Discrete-Time Integrator1/1
  Switch/1 -> Add3/1
  Sign/1 -> Switch/2
  Product/1 -> Sign/1
  Error/1 -> C/1, Gain1/1, Product/1, Gain/1, Derivation/1(E)
  C/1 -> Add1/2

== system MRAS_SMC_SFOC_1_5KW_15May21/FOC_1.5kW/Subsystem3/Flux Calculation2 ==
  Id : Inport
  Discrete Tranfer Function1 : Subsystem  mask(First Order Low Pass Filter (Discrete)){T=Tr, Ts=Tsim}
      mask prompts: T "Time constant T (s) :"; Ts "Time step (s)"
      mask help: H(s)=1/(1+T.s)
      mask init:
      | X=[0 1 2 3 4];
      |  Y=[-2 -2 -3 -4 -4];
      |  str=sprintf('\nH=1/(1+T.s)\n T= %g s\n\n\n',T);
      | num=1;
      | den=[T 1];
      | 
      | % discrete transfer function
      | % descending powers of z
      | numd= Ts/T;
      | dend=[ 1  (Ts-T)/T];
      mask Display:
      | plot(X,Y);
      | disp(str);
  M1 : Gain  Gain=M  SaturateOnIntegerOverflow=on  OutDataTypeStr=Inherit: Same as input  ParamDataTypeStr=Inherit: Same as input
  Phir : Outport
  wires:
  Id/1 -> Discrete Tranfer Function1/1(In)
  M1/1 -> Phir/1
  Discrete Tranfer Function1/1(Out) -> M1/1

== system MRAS_SMC_SFOC_1_5KW_15May21/FOC_1.5kW/Subsystem3/Subsystem1 ==
  Iabc : Inport
  Matrice2 : StateSpace  A=[]  B=[]  C=[]  D=K  InitialCondition=0  mask(Matrix Gain){K=T3_2}
      mask prompts: K "Gain matrix:"
      mask help: Matrix Gain.
      mask Help: Multiplies input vector by entered matrix to produce output vector (y=Au).
      mask Display: disp('K')
  alfa-beta : Outport
  wires:
  Iabc/1 -> Matrice2/1
  Matrice2/1 -> alfa-beta/1

== system MRAS_SMC_SFOC_1_5KW_15May21/FOC_1.5kW/Subsystem3/Teta Calculation2 ==
  Iq : Inport
  Phir : Inport  Port=2
  wm : Inport  Port=3
  Fcn : Fcn  Expr=M*u(1)/(u(2)*Tr+1e-12)
  Gain2 : Gain  SaturateOnIntegerOverflow=on  OutDataTypeStr=Inherit: Same as input  ParamDataTypeStr=Inherit: Same as input
  Kf1 : Gain  Gain=Npole  SaturateOnIntegerOverflow=on  OutDataTypeStr=Inherit: Same as input  ParamDataTypeStr=Inherit: Same as input
  Kf2 : Gain  Gain=2*pi/60  SaturateOnIntegerOverflow=on  OutDataTypeStr=Inherit: Same as input  ParamDataTypeStr=Inherit: Same as input
  Mux : Mux  Inputs=2
  Scope : Scope
  Sum : Sum  SaturateOnIntegerOverflow=on  InputSameDT=on  OutDataTypeStr=Inherit: Same as first input
  ws : Outport  InitialOutput=0
  tag scope: wsl=global
  wires:
  Kf1/1 -> Kf2/1
  Mux/1 -> Fcn/1
  Iq/1 -> Mux/1
  Phir/1 -> Scope/1, Mux/2
  Fcn/1 -> Gain2/1
  wm/1 -> Kf1/1
  Sum/1 -> ws/1
  Kf2/1 -> Sum/2
  Gain2/1 -> [wsl], Sum/1

== system MRAS_SMC_SFOC_1_5KW_15May21/FOC_1.5kW/Subsystem3/alfa_beta to dq2 ==
  Tetas : Inport
  Is_alfa,beta : Inport  Port=2
  Fcn : Fcn  Expr=sin(u)
  Fcn1 : Fcn  Expr=cos(u)
  Gain : Gain  OutDataTypeStr=Inherit: Same as input  ParamDataTypeStr=Inherit: Same as input
  Gain1 : Gain  OutDataTypeStr=Inherit: Same as input  ParamDataTypeStr=Inherit: Same as input
  Mux : Mux  Inputs=[1 1 2]
  id : Fcn  Expr=u[1]*u[3]+u[2]*u[4]
  iq : Fcn  Expr=-u[2]*u[3]+u[1]*u[4]
  Isq : Outport  InitialOutput=0
  Isd : Outport  Port=2  InitialOutput=0
  wires:
  Mux/1 -> iq/1, id/1
  Fcn/1 -> Mux/2
  Fcn1/1 -> Mux/1
  Is_alfa,beta/1 -> Mux/3
  Gain1/1 -> Isq/1
  Gain/1 -> Isd/1
  id/1 -> Gain/1
  iq/1 -> Gain1/1
  Tetas/1 -> Fcn/1, Fcn1/1

== system MRAS_SMC_SFOC_1_5KW_15May21/FOC_1.5kW/Subsystem5/d-Current controller ==
  Error Isd : Inport
  Add1 : Sum
  Discrete-Time Integrator : DiscreteIntegrator  InitialConditionSetting=State (most efficient)  SampleTime=Tsim  LimitOutput=on  UpperSaturationLimit=400  LowerSaturationLimit=-400  ICPrevOutput=DiscIntNeverNeededParam  ICPrevScaledInput=DiscIntNeverNeededParam
  Gain : Gain  Gain=5000
  Gain1 : Gain  Gain=50
  Vsd* : Outport
  wires:
  Gain1/1 -> Add1/2
  Gain/1 -> Discrete-Time Integrator/1
  Add1/1 -> Vsd*/1
  Discrete-Time Integrator/1 -> Add1/1
  Error Isd/1 -> Gain1/1, Gain/1

== system MRAS_SMC_SFOC_1_5KW_15May21/FOC_1.5kW/Subsystem9/q-Current controller ==
  Error Isq : Inport
  Add1 : Sum
  Discrete-Time Integrator : DiscreteIntegrator  InitialConditionSetting=State (most efficient)  SampleTime=Tsim  LimitOutput=on  UpperSaturationLimit=400  LowerSaturationLimit=-400  ICPrevOutput=DiscIntNeverNeededParam  ICPrevScaledInput=DiscIntNeverNeededParam
  Gain : Gain  Gain=5000
  Gain1 : Gain  Gain=50
  Vsq* : Outport
  wires:
  Gain1/1 -> Add1/2
  Gain/1 -> Discrete-Time Integrator/1
  Add1/1 -> Vsq*/1
  Discrete-Time Integrator/1 -> Add1/1
  Error Isq/1 -> Gain1/1, Gain/1

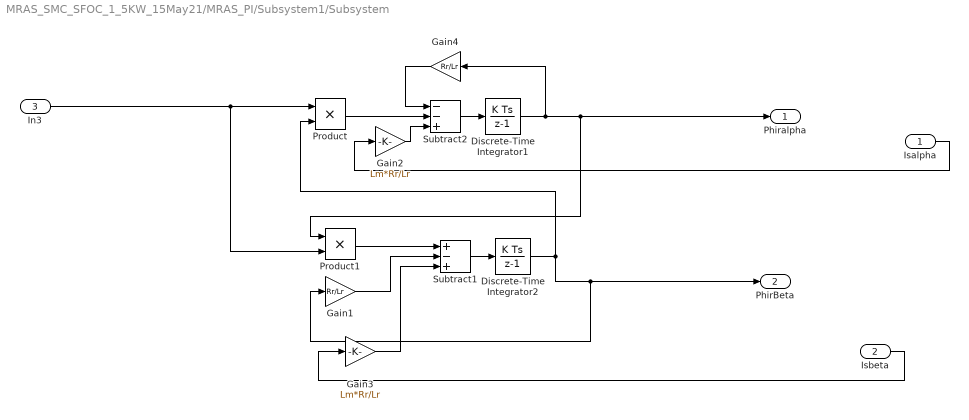
== system MRAS_SMC_SFOC_1_5KW_15May21/MRAS_PI/Subsystem1/Subsystem ==
  Isalpha : Inport
  Isbeta : Inport  Port=2
  In3 : Inport  Port=3
  Discrete-Time Integrator1 : DiscreteIntegrator  InitialConditionSetting=State (most efficient)  SampleTime=Tsim  ICPrevOutput=DiscIntNeverNeededParam  ICPrevScaledInput=DiscIntNeverNeededParam
  Discrete-Time Integrator2 : DiscreteIntegrator  InitialConditionSetting=State (most efficient)  SampleTime=Tsim  ICPrevOutput=DiscIntNeverNeededParam  ICPrevScaledInput=DiscIntNeverNeededParam
  Gain1 : Gain  Gain=Rr/Lr
  Gain2 : Gain  Gain=Lm*Rr/Lr
  Gain3 : Gain  Gain=Lm*Rr/Lr
  Gain4 : Gain  Gain=Rr/Lr
  Product : Product  RndMeth=Zero
  Product1 : Product  RndMeth=Zero
  Subtract1 : Sum  Inputs=+-+
  Subtract2 : Sum  Inputs=--+
  Phiralpha : Outport
  PhirBeta : Outport  Port=2
  wires:
  Gain1/1 -> Subtract1/2
  Gain4/1 -> Subtract2/1
  Product1/1 -> Subtract1/1
  Subtract2/1 -> Discrete-Time Integrator1/1
  Isbeta/1 -> Gain3/1
  Gain3/1 -> Subtract1/3
  Discrete-Time Integrator2/1 -> PhirBeta/1, Gain1/1, Product/2
  Isalpha/1 -> Gain2/1
  Discrete-Time Integrator1/1 -> Gain4/1, Phiralpha/1, Product1/1
  Subtract1/1 -> Discrete-Time Integrator2/1
  Gain2/1 -> Subtract2/3
  Product/1 -> Subtract2/2
  In3/1 -> Product1/2, Product/1

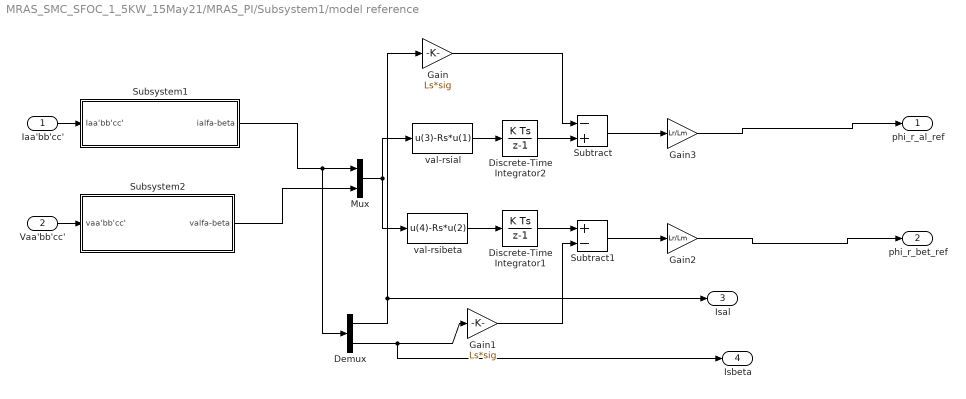
== system MRAS_SMC_SFOC_1_5KW_15May21/MRAS_PI/Subsystem1/model reference ==
  Iaa'bb'cc' : Inport
  Vaa'bb'cc' : Inport  Port=2
  Demux : Demux  Outputs=2
  Discrete-Time Integrator1 : DiscreteIntegrator  InitialConditionSetting=State (most efficient)  SampleTime=Tsim  ICPrevOutput=DiscIntNeverNeededParam  ICPrevScaledInput=DiscIntNeverNeededParam
  Discrete-Time Integrator2 : DiscreteIntegrator  InitialConditionSetting=State (most efficient)  SampleTime=Tsim  ICPrevOutput=DiscIntNeverNeededParam  ICPrevScaledInput=DiscIntNeverNeededParam
  Gain : Gain  Gain=Ls*sig
  Gain1 : Gain  Gain=Ls*sig
  Gain2 : Gain  Gain=Lr/Lm
  Gain3 : Gain  Gain=Lr/Lm
  Mux : Mux  Inputs=[2 2]
  Subsystem1 : Subsystem
  Subsystem2 : Subsystem
  Subtract : Sum  Inputs=-+
  Subtract1 : Sum  Inputs=+-
  val-rsial : Fcn  Expr=u(3)-Rs*u(1)
  val-rsibeta : Fcn  Expr=u(4)-Rs*u(2)
  phi_r_al_ref : Outport
  phi_r_bet_ref : Outport  Port=2
  Isal : Outport  Port=3
  Isbeta : Outport  Port=4
  wires:
  Gain2/1 -> phi_r_bet_ref/1
  Gain3/1 -> phi_r_al_ref/1
  Vaa'bb'cc'/1 -> Subsystem2/1(vaa'bb'cc')
  Iaa'bb'cc'/1 -> Subsystem1/1(Iaa'bb'cc')
  Subtract/1 -> Gain3/1
  Subtract1/1 -> Gain2/1
  Gain1/1 -> Subtract1/2
  Demux/2 -> Gain1/1, Isbeta/1
  Gain/1 -> Subtract/1
  Demux/1 -> Gain/1, Isal/1
  Discrete-Time Integrator1/1 -> Subtract1/1
  Discrete-Time Integrator2/1 -> Subtract/2
  val-rsibeta/1 -> Discrete-Time Integrator1/1
  val-rsial/1 -> Discrete-Time Integrator2/1
  Mux/1 -> val-rsibeta/1, val-rsial/1
  Subsystem2/1(valfa-beta) -> Mux/2
  Subsystem1/1(ialfa-beta) -> Demux/1, Mux/1

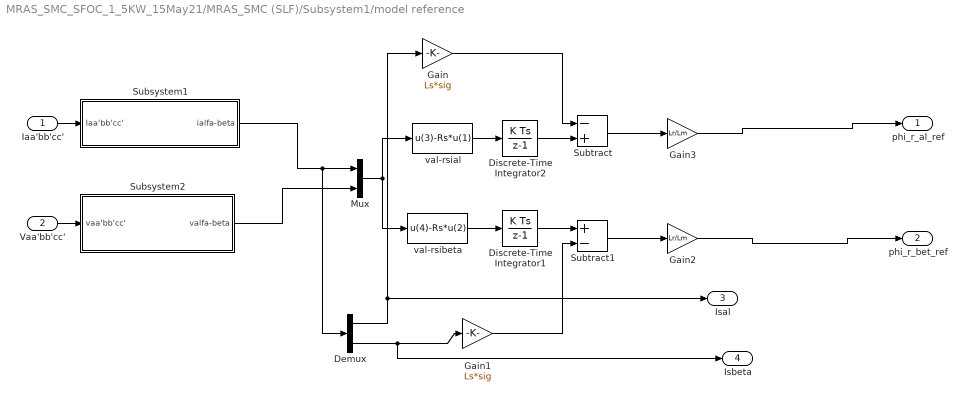
== system MRAS_SMC_SFOC_1_5KW_15May21/MRAS_SMC (SLF)/Subsystem1/model reference ==
  Iaa'bb'cc' : Inport
  Vaa'bb'cc' : Inport  Port=2
  Demux : Demux  Outputs=2
  Discrete-Time Integrator1 : DiscreteIntegrator  InitialConditionSetting=State (most efficient)  SampleTime=Tsim  ICPrevOutput=DiscIntNeverNeededParam  ICPrevScaledInput=DiscIntNeverNeededParam
  Discrete-Time Integrator2 : DiscreteIntegrator  InitialConditionSetting=State (most efficient)  SampleTime=Tsim  ICPrevOutput=DiscIntNeverNeededParam  ICPrevScaledInput=DiscIntNeverNeededParam
  Gain : Gain  Gain=Ls*sig
  Gain1 : Gain  Gain=Ls*sig
  Gain2 : Gain  Gain=Lr/Lm
  Gain3 : Gain  Gain=Lr/Lm
  Mux : Mux  Inputs=[2 2]
  Subsystem1 : Subsystem
  Subsystem2 : Subsystem
  Subtract : Sum  Inputs=-+
  Subtract1 : Sum  Inputs=+-
  val-rsial : Fcn  Expr=u(3)-Rs*u(1)
  val-rsibeta : Fcn  Expr=u(4)-Rs*u(2)
  phi_r_al_ref : Outport
  phi_r_bet_ref : Outport  Port=2
  Isal : Outport  Port=3
  Isbeta : Outport  Port=4
  wires:
  Subsystem1/1(ialfa-beta) -> Mux/1, Demux/1
  Subsystem2/1(valfa-beta) -> Mux/2
  Mux/1 -> val-rsial/1, val-rsibeta/1
  val-rsial/1 -> Discrete-Time Integrator2/1
  val-rsibeta/1 -> Discrete-Time Integrator1/1
  Discrete-Time Integrator2/1 -> Subtract/2
  Discrete-Time Integrator1/1 -> Subtract1/1
  Demux/1 -> Isal/1, Gain/1
  Gain/1 -> Subtract/1
  Demux/2 -> Isbeta/1, Gain1/1
  Gain1/1 -> Subtract1/2
  Subtract1/1 -> Gain2/1
  Subtract/1 -> Gain3/1
  Iaa'bb'cc'/1 -> Subsystem1/1(Iaa'bb'cc')
  Vaa'bb'cc'/1 -> Subsystem2/1(vaa'bb'cc')
  Gain3/1 -> phi_r_al_ref/1
  Gain2/1 -> phi_r_bet_ref/1

== system MRAS_SMC_SFOC_1_5KW_15May21/MRAS_SMC (SLF)/Subsystem6/Derivation ==
  E : Inport
  Add2 : Sum  Inputs=+-
  Delay : Delay  DelayLength=1  SampleTime=Tsim
  Gain3 : Gain  Gain=1/Tsim
  dE/dt : Outport
  wires:
  Add2/1 -> Gain3/1
  E/1 -> Add2/1, Delay/1
  Delay/1 -> Add2/2
  Gain3/1 -> dE/dt/1

== system MRAS_SMC_SFOC_1_5KW_15May21/FOC_1.5kW/Subsystem3/Flux Calculation2/Discrete Tranfer Function1 ==
  In : Inport
  Discrete Transfer Fcn : DiscreteTransferFcn  Numerator=numd  Denominator=dend  SampleTime=Ts
  Out : Outport  InitialOutput=0
  wires:
  Discrete Transfer Fcn/1 -> Out/1
  In/1 -> Discrete Transfer Fcn/1

== system MRAS_SMC_SFOC_1_5KW_15May21/MRAS_PI/Subsystem1/model reference/Subsystem1 ==
  Iaa'bb'cc' : Inport
  Matrice2 : StateSpace  A=[]  B=[]  C=[]  D=K  InitialCondition=0  mask(Matrix Gain){K=T3_2}
      mask prompts: K "Gain matrix:"
      mask help: Matrix Gain.
      mask Help: Multiplies input vector by entered matrix to produce output vector (y=Au).
      mask Display: disp('K')
  ialfa-beta : Outport
  wires:
  Matrice2/1 -> ialfa-beta/1
  Iaa'bb'cc'/1 -> Matrice2/1

== system MRAS_SMC_SFOC_1_5KW_15May21/MRAS_PI/Subsystem1/model reference/Subsystem2 ==
  vaa'bb'cc' : Inport
  Matrice2 : StateSpace  A=[]  B=[]  C=[]  D=K  InitialCondition=0  mask(Matrix Gain){K=T3_2}
      mask prompts: K "Gain matrix:"
      mask help: Matrix Gain.
      mask Help: Multiplies input vector by entered matrix to produce output vector (y=Au).
      mask Display: disp('K')
  valfa-beta : Outport
  wires:
  Matrice2/1 -> valfa-beta/1
  vaa'bb'cc'/1 -> Matrice2/1

== system MRAS_SMC_SFOC_1_5KW_15May21/MRAS_SMC (SLF)/Subsystem1/model reference/Subsystem1 ==
  Iaa'bb'cc' : Inport
  Matrice2 : StateSpace  A=[]  B=[]  C=[]  D=K  InitialCondition=0  mask(Matrix Gain){K=T3_2}
      mask prompts: K "Gain matrix:"
      mask help: Matrix Gain.
      mask Help: Multiplies input vector by entered matrix to produce output vector (y=Au).
      mask Display: disp('K')
  ialfa-beta : Outport
  wires:
  Iaa'bb'cc'/1 -> Matrice2/1
  Matrice2/1 -> ialfa-beta/1

== system MRAS_SMC_SFOC_1_5KW_15May21/MRAS_SMC (SLF)/Subsystem1/model reference/Subsystem2 ==
  vaa'bb'cc' : Inport
  Matrice2 : StateSpace  A=[]  B=[]  C=[]  D=K  InitialCondition=0  mask(Matrix Gain){K=T3_2}
      mask prompts: K "Gain matrix:"
      mask help: Matrix Gain.
      mask Help: Multiplies input vector by entered matrix to produce output vector (y=Au).
      mask Display: disp('K')
  valfa-beta : Outport
  wires:
  vaa'bb'cc'/1 -> Matrice2/1
  Matrice2/1 -> valfa-beta/1
